simulink model "AAI"  (R2022a)
settings: Solver=FixedStepAuto  StartTime=0.0  StopTime=10.0  FixedStep=1e-3  RelTol=1e-3  EnableMultiTasking=on
undefined symbols (not defined in the file): D0, D10, D11, D13, D2, D4, D5, D6, D8, D9, PTA0, PTA2, PTB23, PTB9, PTC16, PTC2, PTC4, PTD0, PTD1, PTD2
libraries: frdmk64flib x10
settings Model: ExtModeTrigDuration=5  Creator=bmile  LastModifiedBy=kemij
settings OptimizationCC: EnhancedBackFolding=on  PassReuseOutputArgsAs=Individual arguments  ZeroExternalMemoryAtStartup=off  ZeroInternalMemoryAtStartup=off  MaxStackSize=64  OptimizeBlockOrder=speed  DifferentSizesBufferReuse=on  OptimizationCustomize=off  EfficientTunableParamExpr=on
settings DebuggingCC: ParameterTunabilityLossMsg=error
settings HardwareCC: ProdBitPerPointer=32  ProdBitPerSizeT=32  ProdBitPerPtrDiffT=32  ProdLargestAtomicInteger=Long  ProdLargestAtomicFloat=Double  ProdWordSize=32  ProdHWDeviceType=ARM Compatible->ARM Cortex
settings SFSimCC: MATLABDynamicMemAlloc=off
settings RTWCC: SystemTargetFile=ert.tlc  HardwareBoard=NXP FRDM-K64F  TLCOptions="-aInlineSetEventsForThisBaseRateFcn=TLC_FALSE -aSuppressMultiTaskScheduler=TLC_FALSE  -aRateBasedStepFcn=0"  TemplateMakefile=ert_default_tmf  Toolchain=GNU Tools for ARM Embedded Processors
settings CodeAppCC: ForceParamTrailComments=on  IgnoreCustomStorageClasses=off  OperatorAnnotations=on  SimulinkDataObjDesc=on  SFDataObjDesc=on  InsertBlockDesc=on
settings ERTTargetCC: ExtModeTransport=4  ExtModeMexFile=sendToCommService

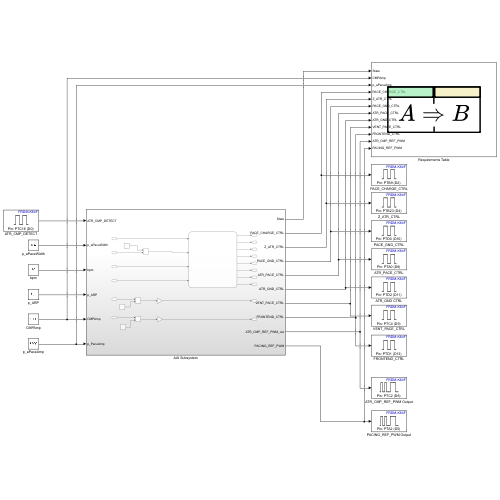
[thumbnail: Simulink's stored preview of the top-level diagram]
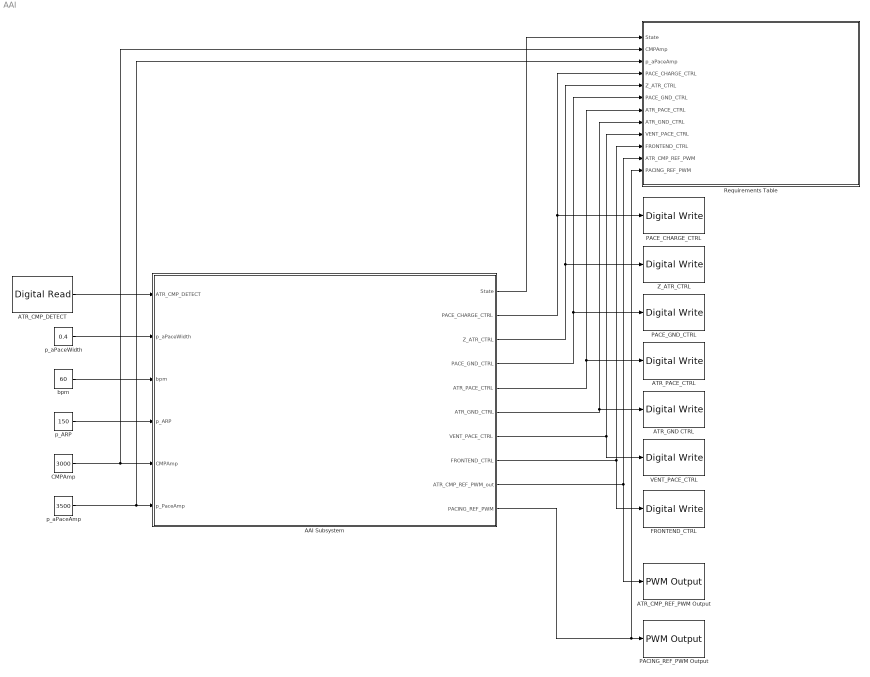
== system AAI ==
  AAI Subsystem : Subsystem
  ATR_CMP_DETECT : frdmk64flib/Digital Read  Whichpin=PTC16 (D0)  SampleTime=-1
  ATR_CMP_REF_PWM Output : frdmk64flib/PWM Output  Whichpin=PTC2 (D6)  InitialFrequency=2000  InitialDutyCycle=0
  ATR_GND CTRL : frdmk64flib/Digital Write  Whichpin=PTD2 (D11)
  ATR_PACE_CTRL : frdmk64flib/Digital Write  Whichpin=PTA0 (D8)
  CMPAmp : Constant  Value=3000
  FRONTEND_CTRL : frdmk64flib/Digital Write  Whichpin=PTD1 (D13)
  PACE_CHARGE_CTRL : frdmk64flib/Digital Write  Whichpin=PTB9 (D2)
  PACE_GND_CTRL : frdmk64flib/Digital Write  Whichpin=PTD0 (D10)
  PACING_REF_PWM Output : frdmk64flib/PWM Output  Whichpin=PTA2 (D5)  InitialFrequency=2000  InitialDutyCycle=0
  Requirements Table : Requirements Table  TreatAsAtomicUnit=on
  VENT_PACE_CTRL : frdmk64flib/Digital Write  Whichpin=PTC4 (D9)
  Z_ATR_CTRL : frdmk64flib/Digital Write  Whichpin=PTB23 (D4)
  bpm : Constant  Value=60
  p_ARP : Constant  Value=150
  p_aPaceAmp : Constant  Value=3500
  p_aPaceWidth : Constant  Value=0.4
  wires:
  AAI Subsystem/4(PACE_GND_CTRL) -> PACE_GND_CTRL/1, Requirements Table/6(PACE_GND_CTRL)
  AAI Subsystem/3(Z_ATR_CTRL) -> Z_ATR_CTRL/1, Requirements Table/5(Z_ATR_CTRL)
  AAI Subsystem/6(ATR_GND_CTRL) -> Requirements Table/8(ATR_GND_CTRL), ATR_GND CTRL/1
  AAI Subsystem/5(ATR_PACE_CTRL) -> ATR_PACE_CTRL/1, Requirements Table/7(ATR_PACE_CTRL)
  p_ARP/1 -> AAI Subsystem/4(p_ARP)
  bpm/1 -> AAI Subsystem/3(bpm)
  ATR_CMP_DETECT/1 -> AAI Subsystem/1(ATR_CMP_DETECT)
  p_aPaceWidth/1 -> AAI Subsystem/2(p_aPaceWidth)
  AAI Subsystem/2(PACE_CHARGE_CTRL) -> Requirements Table/4(PACE_CHARGE_CTRL), PACE_CHARGE_CTRL/1
  AAI Subsystem/8(FRONTEND_CTRL) -> FRONTEND_CTRL/1, Requirements Table/10(FRONTEND_CTRL)
  AAI Subsystem/9(ATR_CMP_REF_PWM_out) -> ATR_CMP_REF_PWM Output/1, Requirements Table/11(ATR_CMP_REF_PWM)
  AAI Subsystem/10(PACING_REF_PWM) -> Requirements Table/12(PACING_REF_PWM), PACING_REF_PWM Output/1
  AAI Subsystem/7(VENT_PACE_CTRL) -> VENT_PACE_CTRL/1, Requirements Table/9(VENT_PACE_CTRL)
  p_aPaceAmp/1 -> Requirements Table/3(p_aPaceAmp), AAI Subsystem/6(p_PaceAmp)
  AAI Subsystem/1(State) -> Requirements Table/1(State)
  CMPAmp/1 -> Requirements Table/2(CMPAmp), AAI Subsystem/5(CMPAmp)

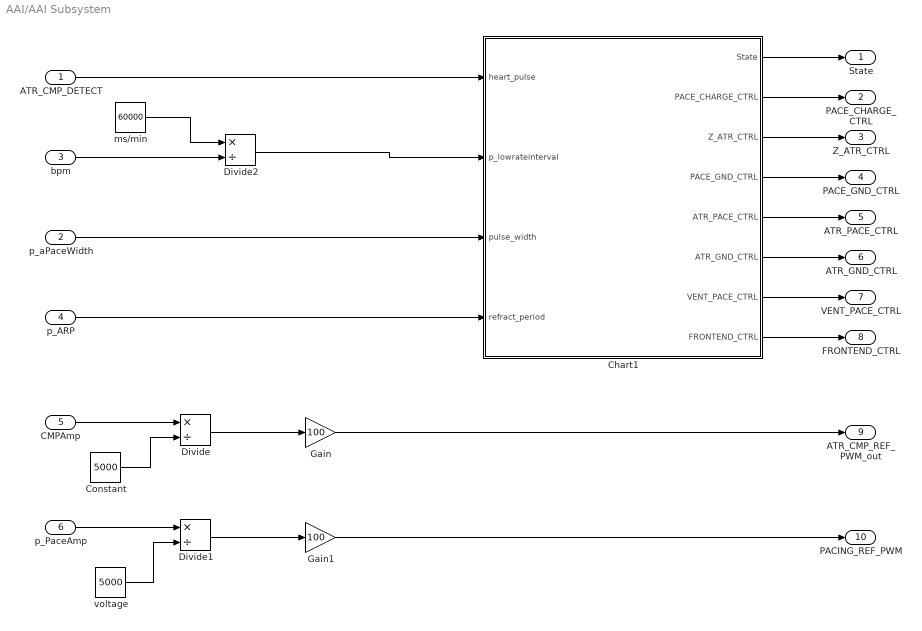
== system AAI/AAI Subsystem ==
  ATR_CMP_DETECT : Inport
  p_aPaceWidth : Inport  Port=2
  bpm : Inport  Port=3
  p_ARP : Inport  Port=4
  CMPAmp : Inport  Port=5
  p_PaceAmp : Inport  Port=6
  Chart1 : Stateflow chart  TreatAsAtomicUnit=on
  Constant : Constant  Value=5000
  Divide : Product  Inputs=*/
  Divide1 : Product  Inputs=*/
  Divide2 : Product  Inputs=*/
  Gain : Gain  Gain=100
  Gain1 : Gain  Gain=100
  ms/min : Constant  Value=60000
  voltage : Constant  Value=5000
  State : Outport
  PACE_CHARGE_CTRL : Outport  Port=2
  Z_ATR_CTRL : Outport  Port=3
  PACE_GND_CTRL : Outport  Port=4
  ATR_PACE_CTRL : Outport  Port=5
  ATR_GND_CTRL : Outport  Port=6
  VENT_PACE_CTRL : Outport  Port=7
  FRONTEND_CTRL : Outport  Port=8
  ATR_CMP_REF_PWM_out : Outport  Port=9
  PACING_REF_PWM : Outport  Port=10
  wires:
  Chart1/8(FRONTEND_CTRL) -> FRONTEND_CTRL/1
  Chart1/7(VENT_PACE_CTRL) -> VENT_PACE_CTRL/1
  Chart1/6(ATR_GND_CTRL) -> ATR_GND_CTRL/1
  Chart1/5(ATR_PACE_CTRL) -> ATR_PACE_CTRL/1
  Chart1/4(PACE_GND_CTRL) -> PACE_GND_CTRL/1
  Chart1/3(Z_ATR_CTRL) -> Z_ATR_CTRL/1
  Chart1/2(PACE_CHARGE_CTRL) -> PACE_CHARGE_CTRL/1
  p_ARP/1 -> Chart1/4(refract_period)
  p_aPaceWidth/1 -> Chart1/3(pulse_width)
  ATR_CMP_DETECT/1 -> Chart1/1(heart_pulse)
  CMPAmp/1 -> Divide/1
  Constant/1 -> Divide/2
  Divide/1 -> Gain/1
  Gain/1 -> ATR_CMP_REF_PWM_out/1
  p_PaceAmp/1 -> Divide1/1
  voltage/1 -> Divide1/2
  Gain1/1 -> PACING_REF_PWM/1
  Divide1/1 -> Gain1/1
  bpm/1 -> Divide2/2
  ms/min/1 -> Divide2/1
  Divide2/1 -> Chart1/2(p_lowrateinterval)
  Chart1/1(State) -> State/1

== stateflow chart AAI/Requirements Table ==
  (default) -> (junction 1073742227)
  (junction 1073742227) -> (junction 1073742228) : {
      | % SF_REQ_REV_07
      | }
  (junction 1073742228) -> (junction 1073742230) : {
      | % HEADER_ASSIGNMENTS
      |
      | }
  (junction 1073742230) -> (junction 1073742232) : {
      | % START_A_4
      | }
  (junction 1073742232) -> (junction 1073742234) : {
      | }
  (junction 1073742234) -> (junction 1073742236)
  (junction 1073742236) -> (junction 1073742238) : {
      | }
  (junction 1073742238) -> (junction 1073742240) : {
      | % END_A_4
      | }
  (junction 1073742240) -> (junction 1073742242) : {
      | % START_R_1
      | }
  (junction 1073742242) -> (junction 1073742244) : {
      | }
  (junction 1073742244) -> (junction 1073742246)
  (junction 1073742246) -> (junction 1073742248) [order 1] : [(((State) == (0))) && (((CMPAmp) == (3000))) && (((p_aPaceAmp) == (3500)))]
  (junction 1073742246) -> (junction 1073742254) [order 2]
  (junction 1073742248) -> (junction 1073742250) : {
      | reqtable_postcondition((((PACE_CHARGE_CTRL) == (true))) && (((Z_ATR_CTRL) == (false))) && (((PACE_GND_CTRL) == (true))) && (((ATR_PACE_CTRL) == (false))) && (((ATR_GND_CTRL) == (true))) && (((VENT_PACE_CTRL) == (false))) && (((FRONTEND_CTRL) == (true))) && (((ATR_CMP_REF_PWM) == (60))) && (((PACING_REF_PWM) == (70))), 'R:1');
      |
      |
      | }
  (junction 1073742250) -> (junction 1073742252) : {
      | }
  (junction 1073742252) -> (junction 1073742254)
  (junction 1073742254) -> (junction 1073742256)
  (junction 1073742256) -> (junction 1073742258) : {
      | % END_R_1
      | }
  (junction 1073742258) -> (junction 1073742260) : {
      | % START_R_7
      | }
  (junction 1073742260) -> (junction 1073742262) : {
      | }
  (junction 1073742262) -> (junction 1073742264)
  (junction 1073742264) -> (junction 1073742266) [order 1] : [(((State) == (1))) && (((CMPAmp) == (3000))) && (((p_aPaceAmp) == (3500)))]
  (junction 1073742264) -> (junction 1073742272) [order 2]
  (junction 1073742266) -> (junction 1073742268) : {
      | reqtable_postcondition((((PACE_CHARGE_CTRL) == (true))) && (((Z_ATR_CTRL) == (false))) && (((PACE_GND_CTRL) == (true))) && (((ATR_PACE_CTRL) == (false))) && (((ATR_GND_CTRL) == (true))) && (((VENT_PACE_CTRL) == (false))) && (((FRONTEND_CTRL) == (true))) && (((ATR_CMP_REF_PWM) == (60))) && (((PACING_REF_PWM) == (70))), 'R:2');
      |
      |
      | }
  (junction 1073742268) -> (junction 1073742270) : {
      | }
  (junction 1073742270) -> (junction 1073742272)
  (junction 1073742272) -> (junction 1073742274)
  (junction 1073742274) -> (junction 1073742276) : {
      | % END_R_7
      | }
  (junction 1073742276) -> (junction 1073742278) : {
      | % START_R_10
      | }
  (junction 1073742278) -> (junction 1073742280) : {
      | }
  (junction 1073742280) -> (junction 1073742282)
  (junction 1073742282) -> (junction 1073742284) [order 1] : [(((State) == (2))) && (((CMPAmp) == (3000))) && (((p_aPaceAmp) == (3500)))]
  (junction 1073742282) -> (junction 1073742290) [order 2]
  (junction 1073742284) -> (junction 1073742286) : {
      | reqtable_postcondition((((PACE_CHARGE_CTRL) == (false))) && (((Z_ATR_CTRL) == (false))) && (((PACE_GND_CTRL) == (true))) && (((ATR_PACE_CTRL) == (true))) && (((ATR_GND_CTRL) == (false))) && (((VENT_PACE_CTRL) == (false))) && (((FRONTEND_CTRL) == (true))) && (((ATR_CMP_REF_PWM) == (60))) && (((PACING_REF_PWM) == (70))), 'R:3');
      |
      |
      | }
  (junction 1073742286) -> (junction 1073742288) : {
      | }
  (junction 1073742288) -> (junction 1073742290)
  (junction 1073742290) -> (junction 1073742292)
  (junction 1073742292) -> (junction 1073742294) : {
      | % END_R_10
      | }
  data: State input; CMPAmp input; p_aPaceAmp input; PACE_CHARGE_CTRL input; Z_ATR_CTRL input; PACE_GND_CTRL input; ATR_PACE_CTRL input; ATR_GND_CTRL input; VENT_PACE_CTRL input; FRONTEND_CTRL input; ATR_CMP_REF_PWM input; PACING_REF_PWM input

== stateflow chart AAI/AAI Subsystem/Chart1 ==
  state Pulse_Sensed
    entry:
    %FRONTEND_CTRL=false
    State = 1
  state Charging_Discharging
    entry:
    ATR_PACE_CTRL = false
    VENT_PACE_CTRL=false
    PACE_CHARGE_CTRL = true
    ATR_GND_CTRL = true
    PACE_GND_CTRL = true
    Z_ATR_CTRL=false
    FRONTEND_CTRL=true
    State = 0
  state Pace_Heart
    entry:
    ATR_PACE_CTRL = true
    PACE_CHARGE_CTRL = false
    PACE_GND_CTRL = true
    ATR_GND_CTRL = false
    State = 2
  Pulse_Sensed -> Charging_Discharging : [after(refract_period,msec)]
  Charging_Discharging -> Pulse_Sensed [order 2] : [heart_pulse == 1]
  (default) -> Charging_Discharging
  Charging_Discharging -> Pace_Heart [order 1] : [after(p_lowrateinterval-pulse_width,msec)]
  Pace_Heart -> Charging_Discharging : after(pulse_width,msec)
  data: State output; heart_pulse input boolean; p_lowrateinterval input; PACE_CHARGE_CTRL output boolean; Z_ATR_CTRL output boolean; PACE_GND_CTRL output boolean; ATR_PACE_CTRL output boolean; ATR_GND_CTRL output boolean; pulse_width input; VENT_PACE_CTRL output boolean; refract_period input; FRONTEND_CTRL output boolean
